simulink model "waypoint_generation_ptCloud_mapdata_filtering_final"  (R2021a)
settings: Solver=ode4  StartTime=0.0  StopTime=500  FixedStep=0.01  RelTol=1e-3  EnableMultiTasking=on
InitFcn:
  | detector = load('ptOPDetector.mat');
  | OPdetector = detector.OPdetector;
undefined symbols (not defined in the file): g, gray, Kd_p, Kd_q, Kd_r, Kd_vx, Kd_vy, Kd_vz, Kff_r, Kff_vx, Kff_vy, Kff_vz, Ki_p, Ki_q, Ki_r, Ki_vx, Ki_vy, Ki_vz, Kp_p, Kp_phi, Kp_psi, Kp_q, Kp_r, Kp_theta, Kp_vx, Kp_vy, Kp_vz, M, pointCloud_center, sigma_motor, w_h
libraries: visiontextngfix x4, sharedtransform x1, shared6dof x1, simulink_extras x1
(part 3 of 3)

== matlab function waypoint_generation_ptCloud_mapdata_filtering_final/MATLAB Function ==
  settings: updateMethod=DISCRETE
  data: current_pos input; pointCloud_current output size=[500000 3]; pointCloud_center input
function pointCloud_current = fcn(current_pos, pointCloud_center)

persistent pointCloud_old block_hz
if isempty(block_hz)
    block_hz = 5;
end
pointCloud_center = double(pointCloud_center);

size_max = 500000;
filtering_distance = 8; %m

pointCloud_new = nan(size_max,3);
pointCloud_current = nan(size_max,3);

% if block_hz ==5
%     block_hz = 0;
    for aaa = 1:numel(pointCloud_center)/3
        if sqrt((pointCloud_center(aaa,1)-current_pos(1))^2+(pointCloud_center(aaa,2)-current_pos(2))^2+(pointCloud_center(aaa,3)-current_pos(3))^2)<filtering_distance
            %         pointCloud_new = cat(1,pointCloud_new,pointCloud_center(aaa,:));
            pointCloud_new(aaa,:) = pointCloud_center(aaa,:);
        end
    end
    
    if isempty(pointCloud_old)
        pointCloud_old = nan(size_max,3);
    end
    
    pointCloud_temp=cat(1,rmmissing(pointCloud_old),rmmissing(pointCloud_new));
    pointCloud_unique = unique(pointCloud_temp,'rows');
    % pointCloud_current=cat(1,cat(1,rmmissing(pointCloud_old),rmmissing(pointCloud_new)),nan(100000-(numel(rmmissing(pointCloud_old))/3+numel(rmmissing(pointCloud_new))/3),3));
    % pointCloud_current=[rmmissing(pointCloud_temp);nan(200000-numel(rmmissing(pointCloud_temp))/3,3)];
    for aaa = 1:numel(pointCloud_unique)/3
        if (~isnan(pointCloud_unique(aaa,1)))&&(~isnan(pointCloud_unique(aaa,2)))&&(~isnan(pointCloud_unique(aaa,3)))
            pointCloud_current(aaa,:)=pointCloud_unique(aaa,:);
        end
    end
    
    
% end

pointCloud_old = pointCloud_current;
% block_hz = block_hz +1;

== matlab function waypoint_generation_ptCloud_mapdata_filtering_final/Quadrotor Dynamics/Translation body -> Earth ==
  data: Ab input; DCM input; Ae output
function Ae = fcn(Ab,DCM)
%#codegen

ax_b = Ab(1);
ay_b = Ab(2);
az_b = Ab(3);

a_b = [ax_b;ay_b;az_b];
Ae = DCM'*a_b;

== matlab function waypoint_generation_ptCloud_mapdata_filtering_final/Position_Controller/Velocity Controller/Acceleration Saturation ==
  data: a_cmd input; a_cmd_sat output; a_norm output
function [a_cmd_sat,a_norm] = fcn(a_cmd)
%#codegen

tilt_max = 35*pi/180; % [rad  ] , tolerant tilt , user define
thr_max  = 11;        % [m/s^2] , tolerant acceleration , user define (90% maximum, 50% hovering)
% thr_max  = 9.8/50 * 90; 

thrust_sp_xy_len = norm([a_cmd(1) a_cmd(2)]);
thrust_xy_max    = abs(a_cmd(3)) * tan(tilt_max);

if thrust_sp_xy_len >= thrust_xy_max
    k =  thrust_xy_max/thrust_sp_xy_len;
    a_cmd_sat = [a_cmd(1)*k ; a_cmd(2)*k ; a_cmd(3)];
else
    a_cmd_sat = a_cmd;
end


if a_cmd_sat(3)/abs(a_cmd_sat(3)) >= 0 
    if abs(a_cmd_sat(3)) >= thr_max

        k  = a_cmd_sat(3) / abs(a_cmd_sat(3));
        a_cmd_sat = [0 ; 0 ; k*thr_max];
    else
        thrust_sp_xy_len_sat = sqrt(a_cmd_sat(1)^2 + a_cmd_sat(2)^2);
        thrust_xy_max_sat    = sqrt(-a_cmd_sat(3)^2 + thr_max^2); 

        if thrust_sp_xy_len_sat >= thrust_xy_max_sat
            k = thrust_xy_max_sat / thrust_sp_xy_len_sat;
            a_cmd_sat = [a_cmd_sat(1)*k ; a_cmd_sat(2)*k ; a_cmd_sat(3)];
        end
    end
else
    a_cmd_sat = [a_cmd_sat(1) ; a_cmd_sat(2) ; 0.00001];
end

a_norm = norm(a_cmd_sat);

== matlab function waypoint_generation_ptCloud_mapdata_filtering_final/Path Guidance/MATLAB Function1 ==
  data: w input; yaw output; x input; y input; z input
function yaw = quat2yaw(w,x,y,z)

euler_angle = quat2eul([w x y z],'ZYX');
yaw = euler_angle(1);
end
